simulink model "BPSK_Demod_FINAL_Prototype_Ready_to_integrate"  (R2013a)
settings: Solver=FixedStepDiscrete  SolverMode=SingleTasking  StartTime=0.0  StopTime=10e3/2400  FixedStep=1/480e3  RelTol=1e-3
undefined symbols (not defined in the file or in its folder): DiscIntNeverNeededParam
libraries: dsparch4 x3, commsynccomp2 x3, dspsigops x3, simulink x2, dspquant2 x1, commchan3 x1, commsink2 x1, commrflib2 x1, commrandsrc2 x1
settings Model: Creator=tibbs2010  LastModifiedBy=tibbs2010
settings DataIOCC: SignalLoggingSaveFormat=ModelDataLogs
settings DebuggingCC: MultiTaskDSMMsg=warning  MultiTaskCondExecSysMsg=none  StrictBusMsg=None
settings RTWCC: IncludeERTFirstTime=on

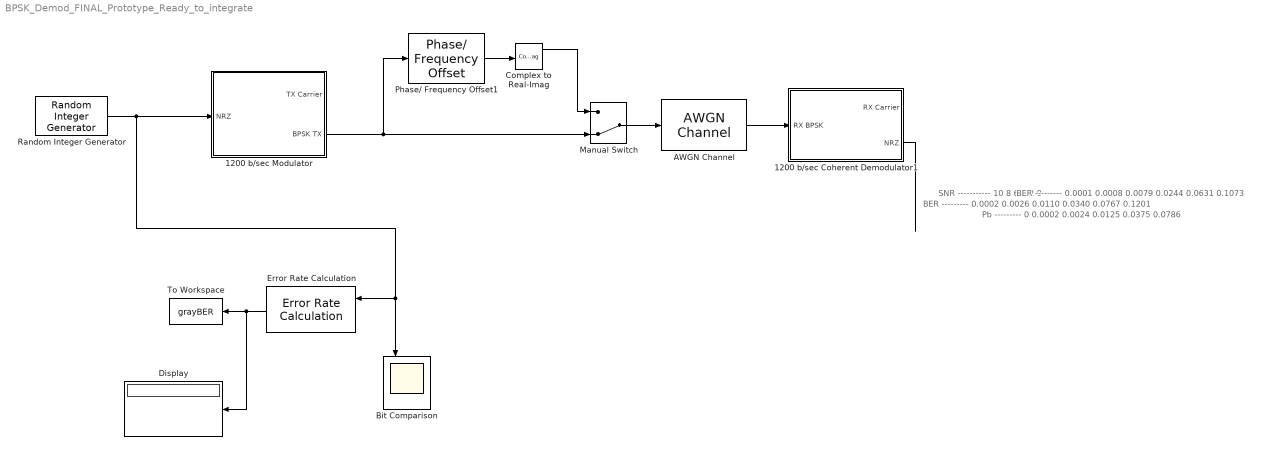
== system BPSK_Demod_FINAL_Prototype_Ready_to_integrate ==
  note: BER
      | ---------
      | 0.0002
      | 0.0026
      | 0.0110
      | 0.0340
      | 0.0767
      | 0.1201
  note: SNR
      | -----------
      |    10
      |      8
      |      6
      |      4
      |      2
      |      0
  note: Pb
      | ---------
      | 0
      | 0.0002
      | 0.0024
      | 0.0125
      | 0.0375
      | 0.0786
  note: BER
      | ---------
      | 0.0001
      | 0.0008
      | 0.0079
      | 0.0244
      | 0.0631
      | 0.1073
  1200 b/sec Modulator : Subsystem
  1200 b/sec Coherent Demodulator1 : Subsystem
  AWGN Channel : commchan3/AWGN Channel  InputProcessing=Columns as channels (frame based)  seed=randseed  noiseMode="Signal to noise ratio  (Eb/No)"  EbNodB=10  EsNodB=10  SNRdB=10  bitsPerSym=1  Ps=12.5  Tsym=1/2400  variance=1
  Bit Comparison : Scope  NumInputPorts=2
      settings: TimeRange=0.008608695652173926  YMin=-0.5~-0.5  YMax=1.5~1.5
  Complex to Real-Imag : ComplexToRealImag
  Display : Display
  Error Rate Calculation : commsink2/Error Rate Calculation  N=2  st_delay=0  cp_mode=Entire frame  subframe=[]  PMode=Port  WsName=grayBER  RsMode2=off  stop=on  numErr=2000  maxBits=10e3
  Manual Switch : ManualSwitch  CurrentSetting=0
  Phase/ Frequency Offset1 : commrflib2/Phase// Frequency Offset  phaseOffset=30  freqPort=off  freqOffset=0
  Random Integer Generator : commrandsrc2/Random Integer Generator  mul=2  seed=randseed  Ts=1/2400  frameBased=off  sampPerFrame=1  orient=off  outDataType=double
  To Workspace : ToWorkspace  VariableName=grayBER  SampleTime=-1  SaveFormat=Timeseries
      settings: MaxDataPoints=1
  wires:
  Error Rate Calculation/1 -> Display/1, To Workspace/1
  1200 b/sec Coherent Demodulator1/2(NRZ) -> ?
  Random Integer Generator/1 -> 1200 b/sec Modulator/1(NRZ), Error Rate Calculation/1, Bit Comparison/1
  1200 b/sec Modulator/2(BPSK TX) -> Manual Switch/2, Phase/ Frequency Offset1/1
  Manual Switch/1 -> AWGN Channel/1
  Phase/ Frequency Offset1/1 -> Complex to Real-Imag/1
  Complex to Real-Imag/1 -> Manual Switch/1
  AWGN Channel/1 -> 1200 b/sec Coherent Demodulator1/1(RX BPSK)

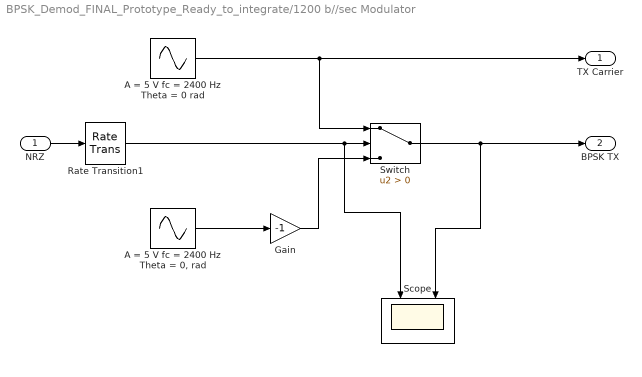
== system BPSK_Demod_FINAL_Prototype_Ready_to_integrate/1200 b//sec Modulator ==
  NRZ : Inport
  A = 5 V fc = 2400 Hz Theta = 0 rad : Sin  Amplitude=5  Frequency=2*pi*4800  Phase=pi/2  SampleTime=1/480e3
  "A = 5 V fc = 2400 Hz Theta = 0, rad" : Sin  Amplitude=5  Frequency=2*pi*4800  Phase=pi/2  Samples=100  SampleTime=1/480e3  Offset=pi
  Gain : Gain  Gain=-1
  Rate Transition1 : RateTransition  OutPortSampleTime=1/480e3
  Scope : Scope  NumInputPorts=2
      settings: TimeRange=0.06  YMin=-1000~-0.5  YMax=1000~1.5  SaveName=ScopeData2
  Switch : Switch  Criteria=u2 > Threshold
  TX Carrier : Outport
  BPSK TX : Outport  Port=2
  wires:
  A = 5 V fc = 2400 Hz Theta = 0 rad/1 -> TX Carrier/1, Switch/1
  "A = 5 V fc = 2400 Hz Theta = 0, rad"/1 -> Gain/1
  Gain/1 -> Switch/3
  NRZ/1 -> Rate Transition1/1
  Switch/1 -> BPSK TX/1, Scope/2
  Rate Transition1/1 -> Scope/1, Switch/2

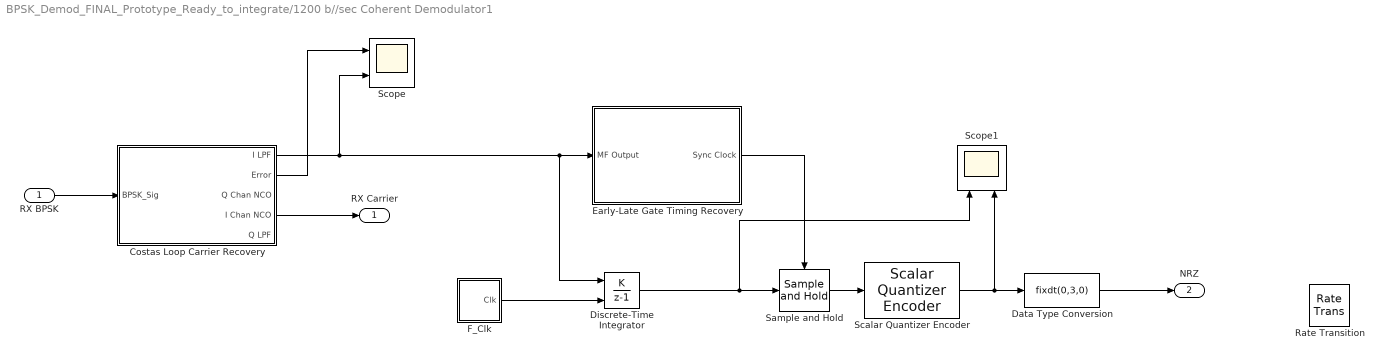
== system BPSK_Demod_FINAL_Prototype_Ready_to_integrate/1200 b//sec Coherent Demodulator1 ==
  RX BPSK : Inport
  Costas Loop Carrier Recovery : Subsystem
  Data Type Conversion : DataTypeConversion  OutDataTypeStr=fixdt(0,3,0)
  Discrete-Time Integrator : DiscreteIntegrator  IntegratorMethod=Accumulation: Forward Euler  ExternalReset=rising  SampleTime=1/480e3  ICPrevOutput=DiscIntNeverNeededParam  ICPrevScaledInput=DiscIntNeverNeededParam
  Early-Late Gate Timing Recovery : Subsystem
  F_Clk : Subsystem
  Rate Transition : RateTransition  OutPortSampleTime=1/1200
  Sample and Hold : dspsigops/Sample and Hold  trig=Rising edge  initCond=0  latchinput=off
  Scalar Quantizer Encoder : dspquant2/Scalar Quantizer Encoder  paramSrc=Specify via dialog  partType=Unbounded  BBoundary=[-250:250]  UBoundary=[-250 -167 -83 0 83 167 250]  SearchMethod=Linear  tieBreakRule=Choose the higher index  outQU=off  outQError=off  codebook=[1.5:9.5]  outStatus=off  invalidin=Clip  idtype=uint8  roundingMode=Floor  overflowMode=off
  Scope : Scope  NumInputPorts=2
      settings: TimeRange=0.0403041825095057  YMin=-30~-12.5  YMax=30~12.5
  Scope1 : Scope  NumInputPorts=2
      settings: TimeRange=0.01093750000000002  YMin=-300~-0.5  YMax=300~1.5  SaveName=ScopeData4
  RX Carrier : Outport
  NRZ : Outport  Port=2
  wires:
  RX BPSK/1 -> Costas Loop Carrier Recovery/1(BPSK_Sig)
  Early-Late Gate Timing Recovery/1(Sync Clock) -> Sample and Hold/Trigger
  Costas Loop Carrier Recovery/1(I LPF) -> Scope/2, Discrete-Time Integrator/1, Early-Late Gate Timing Recovery/1(MF Output)
  Costas Loop Carrier Recovery/2(Error) -> Scope/1
  Discrete-Time Integrator/1 -> Scope1/1, Sample and Hold/1
  F_Clk/1(Clk) -> Discrete-Time Integrator/2
  Costas Loop Carrier Recovery/4(I Chan NCO) -> RX Carrier/1
  Sample and Hold/1 -> Scalar Quantizer Encoder/1
  Scalar Quantizer Encoder/1 -> Data Type Conversion/1, Scope1/2
  Data Type Conversion/1 -> NRZ/1

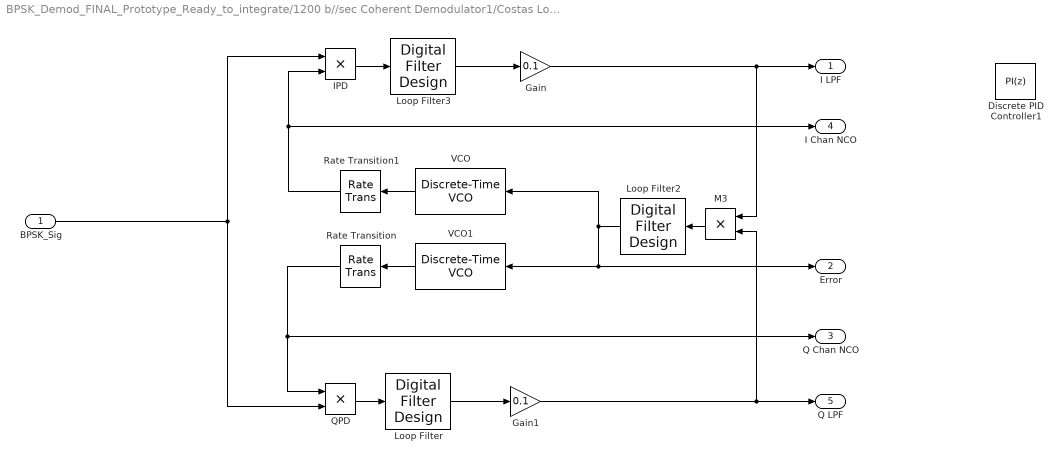
== system BPSK_Demod_FINAL_Prototype_Ready_to_integrate/1200 b//sec Coherent Demodulator1/Costas Loop Carrier Recovery ==
  BPSK_Sig : Inport
  Discrete PID Controller1 : simulink/Continuous/PID Controller  Controller=PI  TimeDomain=Discrete-time  SampleTime=1/480e3  IntegratorMethod=Forward Euler  FilterMethod=Forward Euler  Form=Parallel  P=0.05  I=0.00075  D=0  N=100  InitialConditionSource=internal  InitialConditionForIntegrator=0  InitialConditionForFilter=0  ExternalReset=none  LimitOutput=off  UpperSaturationLimit=inf  LowerSaturationLimit=-inf  LinearizeAsGain=off  AntiWindupMode=none  Kb=1  TrackingMode=off  Kt=1  PParamMin=[]  PParamMax=[]  IParamMin=[]  IParamMax=[]  DParamMin=[]  DParamMax=[]  NParamMin=[]  NParamMax=[]  KbParamMin=[]  KbParamMax=[]  KtParamMin=[]  KtParamMax=[]  POutMin=[]  POutMax=[]  IOutMin=[]  IOutMax=[]  DOutMin=[]  DOutMax=[]  NOutMin=[]  NOutMax=[]  KbOutMin=[]  KbOutMax=[]  KtOutMin=[]  KtOutMax=[]  IntegratorOutMin=[]  IntegratorOutMax=[]  FilterOutMin=[]  FilterOutMax=[]  SumOutMin=[]  SumOutMax=[]  SumI1OutMin=[]  SumI1OutMax=[]  SumI2OutMin=[]  SumI2OutMax=[]  SumI3OutMin=[]  SumI3OutMax=[]  SumDOutMin=[]  SumDOutMax=[]  SaturationOutMin=[]  SaturationOutMax=[]  IntegratorContinuousStateAttributes=''  IntegratorStateMustResolveToSignalObject=off  IntegratorRTWStateStorageClass=Auto  FilterContinuousStateAttributes=''  FilterStateMustResolveToSignalObject=off  FilterRTWStateStorageClass=Auto
  Gain : Gain  Gain=0.1
  Gain1 : Gain  Gain=0.1
  IPD : Product  SampleTime=1/480e3
  Loop Filter : dsparch4/Digital Filter Design  mwdsp_browser_bugfix_var=off
  Loop Filter2 : dsparch4/Digital Filter Design  mwdsp_browser_bugfix_var=off
  Loop Filter3 : dsparch4/Digital Filter Design  mwdsp_browser_bugfix_var=off
  M3 : Product  SampleTime=1/480e3
  QPD : Product  SampleTime=1/480e3
  Rate Transition : RateTransition  OutPortSampleTime=1/480e3
  Rate Transition1 : RateTransition  OutPortSampleTime=1/480e3
  VCO : commsynccomp2/Discrete-Time VCO  Ac=5  Fc=4800  Kc=0.5  Ph=0  ts=1/480e3
  VCO1 : commsynccomp2/Discrete-Time VCO  Ac=5  Fc=4800  Kc=0.5  Ph=pi/2  ts=1/480e3
  I LPF : Outport
  Error : Outport  Port=2
  Q Chan NCO : Outport  Port=3
  I Chan NCO : Outport  Port=4
  Q LPF : Outport  Port=5
  wires:
  VCO/1 -> Rate Transition1/1
  VCO1/1 -> Rate Transition/1
  Rate Transition/1 -> QPD/1, Q Chan NCO/1
  Rate Transition1/1 -> IPD/2, I Chan NCO/1
  QPD/1 -> Loop Filter/1
  IPD/1 -> Loop Filter3/1
  BPSK_Sig/1 -> IPD/1, QPD/2
  Loop Filter/1 -> Gain1/1
  Loop Filter3/1 -> Gain/1
  M3/1 -> Loop Filter2/1
  Loop Filter2/1 -> VCO/1, Error/1, VCO1/1
  Gain/1 -> I LPF/1, M3/1
  Gain1/1 -> Q LPF/1, M3/2

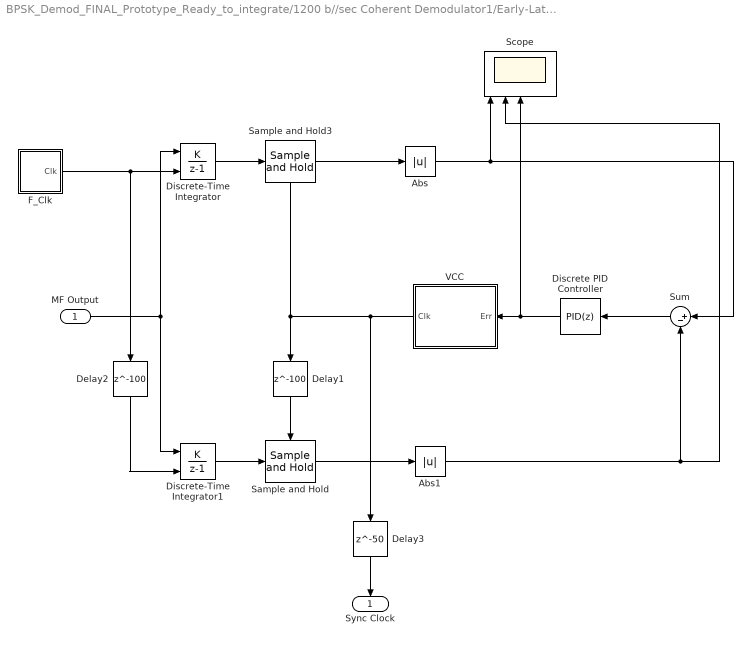
== system BPSK_Demod_FINAL_Prototype_Ready_to_integrate/1200 b//sec Coherent Demodulator1/Early-Late Gate Timing Recovery ==
  MF Output : Inport
  Abs : Abs
  Abs1 : Abs
  Delay1 : Delay  DelayLength=100  InitialCondition=0
  Delay2 : Delay  DelayLength=100  InitialCondition=0
  Delay3 : Delay  DelayLength=50  InitialCondition=0
  Discrete PID Controller : simulink/Continuous/PID Controller  Controller=PID  TimeDomain=Discrete-time  SampleTime=1/480e3  IntegratorMethod=Forward Euler  FilterMethod=Forward Euler  Form=Parallel  P=0.1  I=0.01  D=0  N=0  InitialConditionSource=internal  InitialConditionForIntegrator=0  InitialConditionForFilter=0  ExternalReset=none  LimitOutput=off  UpperSaturationLimit=inf  LowerSaturationLimit=-inf  LinearizeAsGain=off  AntiWindupMode=none  Kb=1  TrackingMode=off  Kt=1  PParamMin=[]  PParamMax=[]  IParamMin=[]  IParamMax=[]  DParamMin=[]  DParamMax=[]  NParamMin=[]  NParamMax=[]  KbParamMin=[]  KbParamMax=[]  KtParamMin=[]  KtParamMax=[]  POutMin=[]  POutMax=[]  IOutMin=[]  IOutMax=[]  DOutMin=[]  DOutMax=[]  NOutMin=[]  NOutMax=[]  KbOutMin=[]  KbOutMax=[]  KtOutMin=[]  KtOutMax=[]  IntegratorOutMin=[]  IntegratorOutMax=[]  FilterOutMin=[]  FilterOutMax=[]  SumOutMin=[]  SumOutMax=[]  SumI1OutMin=[]  SumI1OutMax=[]  SumI2OutMin=[]  SumI2OutMax=[]  SumI3OutMin=[]  SumI3OutMax=[]  SumDOutMin=[]  SumDOutMax=[]  SaturationOutMin=[]  SaturationOutMax=[]  IntegratorContinuousStateAttributes=''  IntegratorStateMustResolveToSignalObject=off  IntegratorRTWStateStorageClass=Auto  FilterContinuousStateAttributes=''  FilterStateMustResolveToSignalObject=off  FilterRTWStateStorageClass=Auto
  Discrete-Time Integrator : DiscreteIntegrator  IntegratorMethod=Accumulation: Forward Euler  ExternalReset=rising  SampleTime=1/480e3  ICPrevOutput=DiscIntNeverNeededParam  ICPrevScaledInput=DiscIntNeverNeededParam
  Discrete-Time Integrator1 : DiscreteIntegrator  IntegratorMethod=Accumulation: Forward Euler  ExternalReset=rising  SampleTime=1/480e3  ICPrevOutput=DiscIntNeverNeededParam  ICPrevScaledInput=DiscIntNeverNeededParam
  F_Clk : Subsystem
  Sample and Hold : dspsigops/Sample and Hold  trig=Rising edge  initCond=0  latchinput=off
  Sample and Hold3 : dspsigops/Sample and Hold  trig=Rising edge  initCond=0  latchinput=off
  Scope : Scope  NumInputPorts=5
      settings: TimeRange=0.06  YMin=110~115~-100~-0.5~-200  YMax=160~160~125~1.5~200  SaveName=ScopeData3
  Sum : Sum  Inputs=|+-
  VCC : Subsystem
  Sync Clock : Outport
  wires:
  Abs1/1 -> Scope/2, Sum/2
  Sample and Hold/1 -> Abs1/1
  Sample and Hold3/1 -> Abs/1
  Sum/1 -> Discrete PID Controller/1
  VCC/1(Clk) -> Delay3/1, Delay1/1, Sample and Hold3/Trigger
  MF Output/1 -> Discrete-Time Integrator/1, Discrete-Time Integrator1/1
  Discrete-Time Integrator/1 -> Sample and Hold3/1
  Discrete-Time Integrator1/1 -> Sample and Hold/1
  Delay2/1 -> Discrete-Time Integrator1/2
  Delay1/1 -> Sample and Hold/Trigger
  Delay3/1 -> Sync Clock/1
  F_Clk/1(Clk) -> Delay2/1, Discrete-Time Integrator/2
  Discrete PID Controller/1 -> Scope/3, VCC/1(Err)
  Abs/1 -> Sum/1, Scope/1

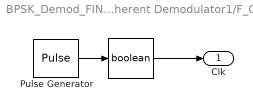
== system BPSK_Demod_FINAL_Prototype_Ready_to_integrate/1200 b//sec Coherent Demodulator1/F_Clk ==
  " " : DataTypeConversion  OutDataTypeStr=boolean
  Pulse Generator : DiscretePulseGenerator  PulseType=Time based  Amplitude=5  Period=1/2400  PulseWidth=50  SampleTime=1/480e3
  Clk : Outport
  wires:
  " "/1 -> Clk/1
  Pulse Generator/1 -> " "/1

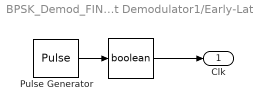
== system BPSK_Demod_FINAL_Prototype_Ready_to_integrate/1200 b//sec Coherent Demodulator1/Early-Late Gate Timing Recovery/F_Clk ==
  " " : DataTypeConversion  OutDataTypeStr=boolean
  Pulse Generator : DiscretePulseGenerator  PulseType=Time based  Amplitude=5  Period=1/2400  PulseWidth=50  SampleTime=1/480e3
  Clk : Outport
  wires:
  " "/1 -> Clk/1
  Pulse Generator/1 -> " "/1

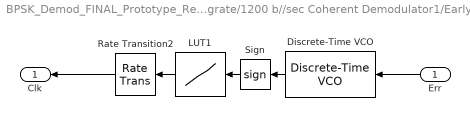
== system BPSK_Demod_FINAL_Prototype_Ready_to_integrate/1200 b//sec Coherent Demodulator1/Early-Late Gate Timing Recovery/VCC ==
  Err : Inport
  Discrete-Time VCO : commsynccomp2/Discrete-Time VCO  Ac=1  Fc=2400  Kc=1  Ph=0  ts=1/480e3
  LUT1 : Lookup_n-D  NumberOfTableDimensions=1  BreakpointsForDimension1=[-1 0 1]  Table=[0 0 1]  RndMeth=Simplest  InputSameDT=on
  Rate Transition2 : RateTransition  OutPortSampleTime=1/480e3
  Sign : Signum
  Clk : Outport
  wires:
  Discrete-Time VCO/1 -> Sign/1
  Err/1 -> Discrete-Time VCO/1
  LUT1/1 -> Rate Transition2/1
  Rate Transition2/1 -> Clk/1
  Sign/1 -> LUT1/1
